simulink model "loaded_motor"  (R2021b)
settings: Solver=VariableStepAuto  StartTime=0.0  StopTime=0.5  RelTol=1e-3
undefined symbols (not defined in the file or in its folder): Km
libraries: cstblocks x3
settings Model: Creator=andre  LastModifiedBy=andre

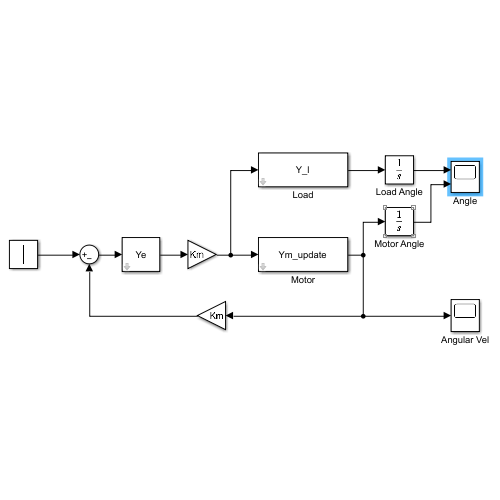
[thumbnail: Simulink's stored preview of the top-level diagram]
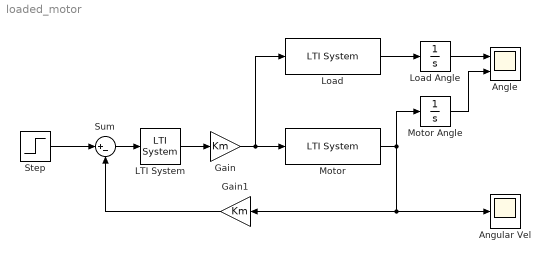
== system loaded_motor ==
  Angle : Scope  NumInputPorts=2
  Angular Vel : Scope
  Gain : Gain  Gain=Km
  Gain1 : Gain  Gain=Km
  LTI System : cstblocks/LTI System  sys=Ye  IC=[]
  Load : cstblocks/LTI System  sys=Y_l  IC=[]
  Load Angle : Integrator
  Motor : cstblocks/LTI System  sys=Ym_update  IC=[]
  Motor Angle : Integrator
  Step : Step  Time=0  After=6  SampleTime=0
  Sum : Sum  Inputs=|+-
  wires:
  LTI System/1 -> Gain/1
  Gain/1 -> Load/1, Motor/1
  Motor/1 -> Gain1/1, Angular Vel/1, Motor Angle/1
  Step/1 -> Sum/1
  Gain1/1 -> Sum/2
  Sum/1 -> LTI System/1
  Load/1 -> Load Angle/1
  Load Angle/1 -> Angle/1
  Motor Angle/1 -> Angle/2
